simulink model "rtwdemo_ratetrans"  (Simulink 7.6)
settings: Solver=FixedStepDiscrete  SolverMode=MultiTasking  StartTime=0.0  StopTime=0.5  FixedStep=1/2000  RelTol=1e-3  AbsTol=1e-6
PreLoadFcn:
  | width = 160;
undefined symbols (not defined in the file or in its folder): DiscIntNeverNeededParam
libraries: rtwdemowidgets x3, simulink x1
Description:
  | Trading Determinism and Data Integrity to Improve System Performance
settings Model: Creator=The MathWorks Inc.  ExtModeTrigMode=oneshot  ExtModeArmWhenConnect=off  ExtModeAutoUpdateStatusClock=off
settings MATStruct: SampleTime=1/2000  Offset=0  Priority=[44.0]
settings DataIOCC: LimitDataPoints=off  SaveOutput=off  SaveTime=off  SignalLoggingName=sigsOut
settings OptimizationCC: InlineParams=on  InlineInvariantSignals=on  StateBitsets=on  DataBitsets=on  UseTempVars=on  EfficientFloat2IntCast=on  EfficientMapNaN2IntZero=off
settings DebuggingCC: CheckExecutionContextPreStartOutputMsg=on  CheckExecutionContextRuntimeOutputMsg=on  SolverPrmCheckMsg=none  InheritedTsInSrcMsg=none  IntegerOverflowMsg=none  UnconnectedInputMsg=none  UnconnectedOutputMsg=none  UnconnectedLineMsg=none  StrictBusMsg=ErrorOnBusTreatedAsVector
settings HardwareCC: ProdIntDivRoundTo=Zero  ProdEndianess=LittleEndian  ProdHWDeviceType=Generic->32-bit Embedded Processor  TargetHWDeviceType=Generic->32-bit Embedded Processor
settings ModelReferenceCC: UpdateModelReferenceTargets=IfOutOfDate
settings RTWCC: TLCOptions=-p0 -aWarnNonSaturatedBlocks=0  GenerateReport=on  RTWVerbose=off  ProcessScript=grt_make_rtw_hook  LaunchReport=on
settings CodeAppCC: ForceParamTrailComments=on
settings GRTTargetCC: TargetFcnLib=ansi_tfl_tmw.mat

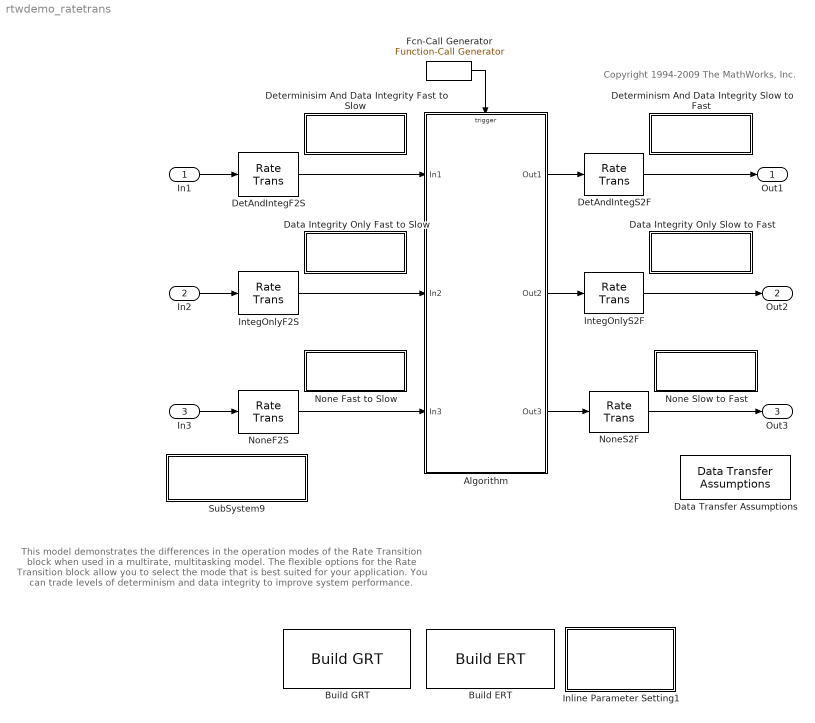
== system rtwdemo_ratetrans ==
  note: This model demonstrates the differences in the operation modes of the Rate Transition
      | block when used in a multirate, multitasking model.  The flexible options for the Rate
      | Transition block allow you to select the mode that is best suited for your application.
      | You can trade levels of determinism and data integrity to improve system performance.
  note: Copyright 1994-2009 The MathWorks, Inc.
  In1 : Inport  OutDataTypeStr=double  PortDimensions=20  SampleTime=1/2000
  In2 : Inport  Port=2  OutDataTypeStr=double  PortDimensions=20  SampleTime=1/2000
  In3 : Inport  Port=3  OutDataTypeStr=double  PortDimensions=20  SampleTime=1/2000
  Algorithm : Subsystem  TreatAsAtomicUnit=on  RTWFcnName=Algorithm  RTWFileName=Algorithm
      settings: RTWFcnNameOpts=User specified  RTWFileNameOpts=User specified
  Build ERT : rtwdemowidgets/Build ERT  SystemSampleTime=-1  attrib_overrides={}
  Build GRT : rtwdemowidgets/Build GRT  SystemSampleTime=-1  attrib_overrides={}
  Data Integrity Only Fast to Slow : Subsystem
      mask Display: disp(['Generated Code\nDescription..','.'])
  Data Integrity Only Slow to Fast : Subsystem
      mask Display: disp(['Generated Code\nDescription..','.'])
  Data Transfer Assumptions : rtwdemowidgets/Data Transfer Assumptions  SystemSampleTime=-1
  DetAndIntegF2S : RateTransition  OutPortSampleTime=1/1000
  DetAndIntegS2F : RateTransition  OutPortSampleTime=1/2000
  Determinisim And Data Integrity Fast to Slow : Subsystem
      mask Display: disp(['Generated Code\nDescription..','.'])
  Determinism And Data Integrity Slow to Fast : Subsystem
      mask Display: disp(['Generated Code\nDescription..','.'])
  Fcn-Call Generator : simulink/Ports & Subsystems/Function-Call Generator  sample_time=1/1000  numberOfIterations=1
  Inline Parameter Setting1 : Subsystem
      settings: OpenFcn=m=get_param(bdroot,'name'); set_param(bdroot, 'SampleTimeColors','on'); eval([m,'([],[],[],''compile'');']); eval([m,'([],[],[],''term'');']); clear m;
      mask Display: disp(sprintf('Display Sample\nTime Colors\n(double-click)'))
  IntegOnlyF2S : RateTransition  Deterministic=off  OutPortSampleTime=1/1000
  IntegOnlyS2F : RateTransition  Deterministic=off  OutPortSampleTime=1/2000
  None Fast to Slow : Subsystem
      mask Display: disp(['Generated Code\nDescription..','.'])
  None Slow to Fast : Subsystem
      mask Display: disp(['Generated Code\nDescription..','.'])
  NoneF2S : RateTransition  Integrity=off  Deterministic=off  OutPortSampleTime=1/1000
  NoneS2F : RateTransition  Integrity=off  Deterministic=off  OutPortSampleTime=1/2000
  SubSystem9 : Subsystem
      mask Display: text(.05,.5,['Rate Transition Block\nModes..','.'])
  Out1 : Outport
  Out2 : Outport  Port=2
  Out3 : Outport  Port=3
  wires:
  IntegOnlyS2F/1 -> Out2/1
  Fcn-Call Generator/1 -> Algorithm/Trigger
  IntegOnlyF2S/1 -> Algorithm/2(In2)
  DetAndIntegF2S/1 -> Algorithm/1(In1)
  Algorithm/1(Out1) -> DetAndIntegS2F/1
  Algorithm/2(Out2) -> IntegOnlyS2F/1
  DetAndIntegS2F/1 -> Out1/1
  NoneF2S/1 -> Algorithm/3(In3)
  Algorithm/3(Out3) -> NoneS2F/1
  NoneS2F/1 -> Out3/1
  In1/1 -> DetAndIntegF2S/1
  In2/1 -> IntegOnlyF2S/1
  In3/1 -> NoneF2S/1

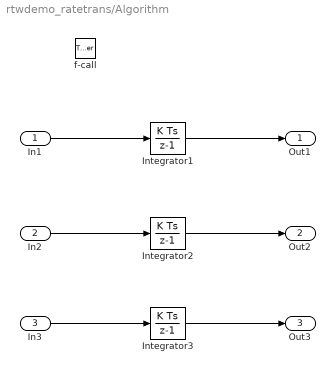
== system rtwdemo_ratetrans/Algorithm ==
  In1 : Inport
  In2 : Inport  Port=2
  In3 : Inport  Port=3
  f-call : TriggerPort  TriggerType=function-call
  Integrator1 : DiscreteIntegrator  InitialConditionMode=State only (most efficient)  SampleTime=-1  SaturateOnIntegerOverflow=on  ICPrevOutput=DiscIntNeverNeededParam  ICPrevScaledInput=DiscIntNeverNeededParam
  Integrator2 : DiscreteIntegrator  InitialConditionMode=State only (most efficient)  SampleTime=-1  SaturateOnIntegerOverflow=on  ICPrevOutput=DiscIntNeverNeededParam  ICPrevScaledInput=DiscIntNeverNeededParam
  Integrator3 : DiscreteIntegrator  InitialConditionMode=State only (most efficient)  SampleTime=-1  SaturateOnIntegerOverflow=on  ICPrevOutput=DiscIntNeverNeededParam  ICPrevScaledInput=DiscIntNeverNeededParam
  Out1 : Outport  InitialOutput=0
  Out2 : Outport  Port=2  InitialOutput=0
  Out3 : Outport  Port=3  InitialOutput=0
  wires:
  In1/1 -> Integrator1/1
  Integrator1/1 -> Out1/1
  In2/1 -> Integrator2/1
  Integrator2/1 -> Out2/1
  In3/1 -> Integrator3/1
  Integrator3/1 -> Out3/1

== system rtwdemo_ratetrans/Data Integrity Only Fast to Slow ==
  note: Data integrity only (fast to slow transition):
      |
      | o The block output is used as a persistent data buffer.
      |
      | o Data is written to buffer during the faster rate context if a flag indicates
      | it not in the process of being read.
      |
      | o The flag is set and data is copied from the buffer to output at the slow
      | rate, the flag is then cleared. This is an additional copy as compared to the
      |  deterministic case.
      |
      | o Data as seen by the slower rate can be from a more recent step of the faster
      | rate than from when the slower rate and faster rate both executed.

== system rtwdemo_ratetrans/Data Integrity Only Slow to Fast ==
  note: Data integrity only (slow to fast transition):
      |
      | o Uses two persistent data buffers, both are internal buffers.
      |
      | o One of the 2 buffers is always copied to the output at faster rate.
      |
      | o One of the 2 buffers is written at the slower rate and during the slower rate
      | context, then the active buffer is switched.
      |
      | o The data as seen by the faster rate can be more recent than for the
      | deterministic case. Specifically, when both the slower and faster rate have
      | their hits, the faster rate will see a previous value from the slower
      | rate. But, subsequent steps for the faster rate may see an updated value (when
      | the slower rate updates the non-active buffer and switches the active buffer
      | flag.

== system rtwdemo_ratetrans/Determinisim And Data Integrity Fast to Slow ==
  note: Determinism and data integrity (fast->slow transition):
      |
      | o The block output is used as a persistent data buffer.
      |
      | o Data is written to output at slower rate but done during the faster rate context
      |
      | o Data as seen by the slower rate is always the value when both the faster and
      | slower rate last executed. Any subsequent steps by the faster rate (and
      | associated data updates) while the slower rate is running are not seen by the
      | slower rate.

== system rtwdemo_ratetrans/Determinism And Data Integrity Slow to Fast ==
  note: Determinism and data integrity (slow to fast transition):
      |
      | o Uses two persistent data buffers, an internal buffer and the blocks output.
      |
      | o The internal buffer is copied to the output at the slower rate but done during
      |  the faster rate context.
      |
      | o The internal buffer is written at the slower rate and during the slower rate context.
      |
      | o The data that Fast rate sees is always delayed, i.e. data is from the
      | previous step of the slow rate code.

== system rtwdemo_ratetrans/Inline Parameter Setting1 ==

== system rtwdemo_ratetrans/None Fast to Slow ==
  note: No code is generated for the Rate Transition block when
      | determinism and data integrity is waived.

== system rtwdemo_ratetrans/None Slow to Fast ==
  note: No code is generated for the Rate Transition block when
      | determinism and data integrity is waived.

== system rtwdemo_ratetrans/SubSystem9 ==
  note: Rate Transition Block Modes of Operation:
      |
      | 1) Ensure data integrity and determinism (DetAndInteg): Data is transferred such
      |    that all data bytes for the signal (including all elements of a wide signal)
      |    are from the same time step. Additionally, it is ensured that the relative
      |    sample time (delay) from which the data is transferred from one rate to
      |    another is always the same. Only ANSI-C code is used, no target specific 'critical
      |    section' protection is needed.
      |
      | 2) Ensure integrity (IntegOnly): Data is transferred such that all data bytes for the
      |    signal (including all elements of a wide signal) are from the same time
      |    step. However, from one transfer of data to the next, the relative sample
      |    time (delay) for which the data is transferred can vary. In this mode, the code to
      |    read/write the data is run more often than in the DetandInt mode. In the
      |    worst case, the delay is equivalent to the DetandInt mode, but the delay can
      |    be less which is important is some applications.  Also, this mode support
      |    data transfers to/from asynchronous rates which the DetandInt mode cannot
      |    support. Only ANSI-C code is used, no target specific 'critical
      |    section' protection is needed.
      |
      | 3) No data consistency operations are performed (None): For this case, the Rate
      |    Transition block does not generated code. This mode is acceptable in
      |    some application where atomic access of scalar data types is guaranteed and
      |    when the relative temporal values of the data is not important. This mode
      |    does not introduce any delay.
